simulink model "untitled"  (R2023a)
settings: Solver=VariableStepAuto  StartTime=0.0  StopTime=10.0  RelTol=1e-3
libraries: ros2lib x2
settings Model: Creator=vinny-desktop-win10  LastModifiedBy=vinny-desktop-win10

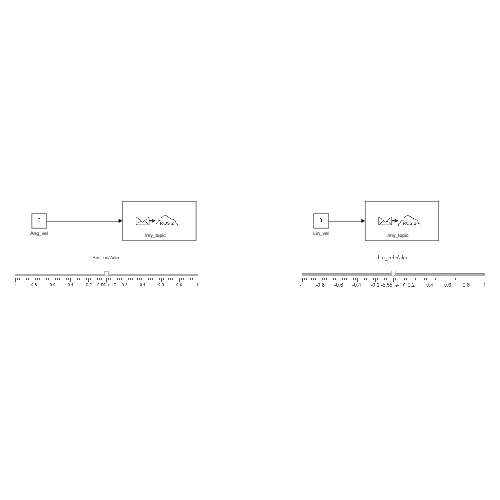
[thumbnail: Simulink's stored preview of the top-level diagram]
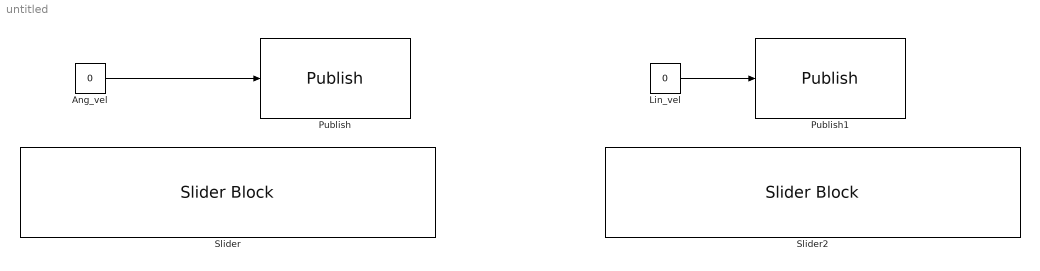
== system untitled ==
  Ang_vel : Constant  Value=0  OutDataTypeStr=int8  LockScale=on
  Lin_vel : Constant  Value=0  OutDataTypeStr=int8  LockScale=on
  Publish : ros2lib/Publish  topicSource=Specify your own  topic=/my_topic  messageType=geometry_msgs/Twist  QOSHistory=Keep last  QOSDepth=1  QOSReliability=Reliable  QOSDurability=Volatile
  Publish1 : ros2lib/Publish  topicSource=Select from ROS network  topic=/my_topic  messageType=geometry_msgs/Point  QOSHistory=Keep last  QOSDepth=1  QOSReliability=Reliable  QOSDurability=Volatile
  Slider : SliderBlock  ScaleMin=-1  ScaleMax=1  TickInterval=0.2
  Slider2 : SliderBlock  ScaleMin=-1  ScaleMax=1  TickInterval=0.2
  wires:
  Ang_vel/1 -> Publish/1
  Lin_vel/1 -> Publish1/1
